simulink model "reverbe2"  (R2019a)
settings: Solver=VariableStepAuto  StartTime=0.0  StopTime=60  RelTol=1e-3
libraries: Librairie x2, dspobslib x1
settings Model: Creator=shse  LastModifiedBy=Ahmed

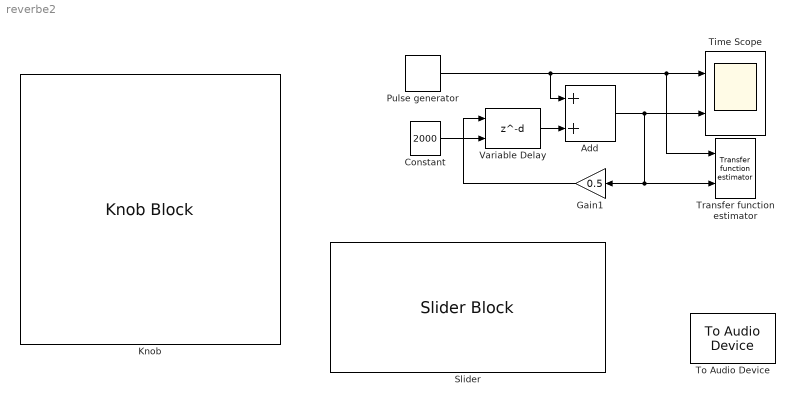
== system reverbe2 ==
  Add : Sum
  Constant : Constant  Value=2000  VectorParams1D=off
  Gain1 : Gain  Gain=0.5
  Knob : KnobBlock  ScaleMax=44100
  Pulse generator : Librairie/Pulse generator  fee=11025  NN=1024
  Slider : SliderBlock  ScaleMax=2
  Time Scope : Scope  NumInputPorts=2
  To Audio Device : dspobslib/To Audio Device  deviceName=Default  inheritSampleRate=on  sampleRate=44100  deviceDatatype=Determine from input data type  autoBufferSize=on  bufferSize=4096  queueDuration=1.0  defaultOutputChannelMapping=on  outputChannelMapping=1:2  outputNumUnderrunSamples=off
      settings: SourceProductName=DSP System Toolbox  SourceProductBaseCode=DS
  Transfer function estimator : Librairie/Transfer function estimator  fee=11025  NN=1024
  Variable Delay : Delay  DelayLengthSource=Input port  DelayLength=1  DelayLengthUpperLimit=5000  PreventDirectFeedthrough=on  RemoveDelayLengthCheckInGeneratedCode=on  InputProcessing=Columns as channels (frame based)
      settings: InputPortMap=u0,p1
  wires:
  Pulse generator/1 -> Transfer function estimator/1, Time Scope/1, Add/1
  Add/1 -> Gain1/1, Transfer function estimator/2, Time Scope/2
  Gain1/1 -> Variable Delay/1
  Variable Delay/1 -> Add/2
  Constant/1 -> Variable Delay/2
